simulink model "mfsk"  (R2015b)
settings: Solver=VariableStepAuto  StartTime=0.0  StopTime=10.0  RelTol=1e-3
libraries: commdigbbndfm2 x2, commchan3 x1, commrandsrc3 x1
settings Model: Creator=Alex  LastModifiedBy=Alex

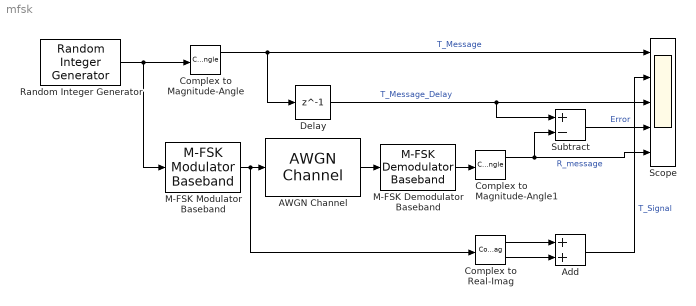
== system mfsk ==
  AWGN Channel : commchan3/AWGN Channel  InputProcessing=Columns as channels (frame based)  seed=67  noiseMode="Signal to noise ratio  (Eb/No)"  EbNodB=10  EsNodB=10  SNRdB=10  bitsPerSym=1  Ps=1  Tsym=1  variance=1
  Add : Sum
  Complex to Magnitude-Angle : ComplexToMagnitudeAngle
  Complex to Magnitude-Angle1 : ComplexToMagnitudeAngle
  Complex to Real-Imag : ComplexToRealImag
  Delay : Delay  DelayLength=1  InitialCondition=0
  M-FSK Demodulator Baseband : commdigbbndfm2/M-FSK Demodulator Baseband  M=8  OutType=Integer  Dec=Gray  freqSep=6  numSamp=17  RateOptions=Enforce single-rate processing  outDataType=double
  M-FSK Modulator Baseband : commdigbbndfm2/M-FSK Modulator Baseband  M=8  InType=Integer  Enc=Gray  freqSep=6  phaseType=Continuous  numSamp=17  RateOptions=Enforce single-rate processing  outDataType=double
  Random Integer Generator : commrandsrc3/Random Integer Generator  SetSize=8  SeedSource=Auto  Seed=0  SampleTime=1  SamplesPerFrame=1  OutputDataType=double  SimulateUsing=Interpreted execution
  Scope : Scope  NumInputPorts=5
  Subtract : Sum  Inputs=+-
  wires:
  Random Integer Generator/1 -> M-FSK Modulator Baseband/1, Complex to Magnitude-Angle/1
  M-FSK Modulator Baseband/1 -> Complex to Real-Imag/1, AWGN Channel/1
  AWGN Channel/1 -> M-FSK Demodulator Baseband/1
  M-FSK Demodulator Baseband/1 -> Complex to Magnitude-Angle1/1
  Complex to Magnitude-Angle/1 -> Delay/1, Scope/1  "T_Message"
  Complex to Magnitude-Angle1/1 -> Scope/5, Subtract/2  "R_message"
  Delay/1 -> Subtract/1, Scope/3  "T_Message_Delay"
  Complex to Real-Imag/1 -> Add/1
  Complex to Real-Imag/2 -> Add/2
  Subtract/1 -> Scope/4  "Error"
  Add/1 -> Scope/2  "T_Signal"
